simulink model "mpc_pendcartPlan.slx"  (R2017a)
settings: Solver=ode45  StartTime=0.0  StopTime=10.0  RelTol=1e-3
values from neighbouring files (symbols this model uses):
  l = 0.35    [lqr_1dof (run this).m]
undefined symbols (not defined in the file or in its folder): I
settings Model: Creator=sansh  LastModifiedBy=rj2318

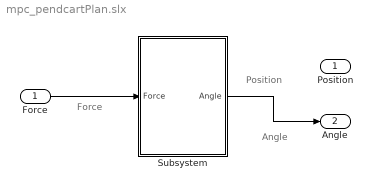
== system mpc_pendcartPlan.slx ==
  note: Angle
  note: Position
  note: Force
  Force : Inport
  Subsystem : Subsystem
  Position : Outport
  Angle : Outport  Port=2
  wires:
  Force/1 -> Subsystem/1(Force)
  ? -> Position/1
  Subsystem/1(Angle) -> Angle/1

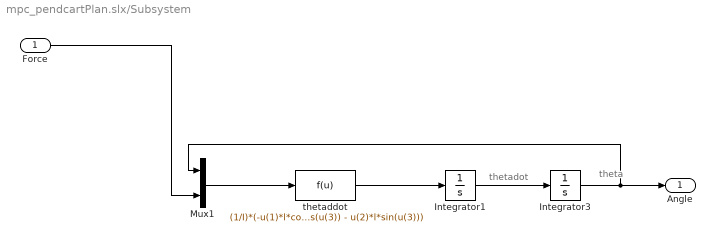
== system mpc_pendcartPlan.slx/Subsystem ==
  note: theta
  note: thetadot
  Force : Inport
  Integrator1 : Integrator  ContinuousStateAttributes='thetadot'
  Integrator3 : Integrator  InitialCondition=pi  ContinuousStateAttributes='theta'
  Mux1 : Mux  Inputs=2
  thetaddot : Fcn  Expr=(1/I)*(-u(1)*l*cos(u(3)) - u(2)*l*sin(u(3)))
  Angle : Outport
  wires:
  Mux1/1 -> thetaddot/1
  thetaddot/1 -> Integrator1/1
  Integrator1/1 -> Integrator3/1
  Integrator3/1 -> Mux1/1, Angle/1
  Force/1 -> Mux1/2
